simulink model "cobem_simulink_alpha1_0"  (R2018a)
settings: Solver=ode4  StartTime=0.0  StopTime=tempo_simu  FixedStep=1e-3  RelTol=1e-3
values from neighbouring files (symbols this model uses):
  Area1 = 3.1416    [clc.mat]    (also in cobem_teste_PSO.m)
  Area2 = 0.0113    [clc.mat]    (also in cobem_teste_PSO.m)
  Area4 = 0.0314    [clc.mat]    (also in cobem_teste_PSO.m)
  Fnom = 60    [clc.mat]    (also in cobem_teste_PSO.m)
  g = 9.81    [clc.mat]    (also in cobem_teste_PSO.m)
  h10 = 0.5    [clc.mat]    (also in cobem_teste_PSO.m)
  h20 = 0.5    [clc.mat]    (also in cobem_teste_PSO.m)
  Hmax = 3    [clc.mat]    (also in cobem_teste_PSO.m)
  Kd = abs(current_position(3,i))    [cobem_teste_PSO.m]
  Ki = abs(current_position(2,i))    [cobem_teste_PSO.m]
  Kp = abs(current_position(1,i))    [cobem_teste_PSO.m]
  pho = 998.23    [clc.mat]    (also in cobem_teste_PSO.m)
  Qe = 31360.39368    [clc.mat]    (also in cobem_teste_PSO.m)
  Rmax = 1    [clc.mat]    (also in cobem_teste_PSO.m)
  t_filtro = 0.0426    [clc.mat]    (also in cobem_teste_PSO.m)
settings Model: Creator=generic-user  LastModifiedBy=generic-user

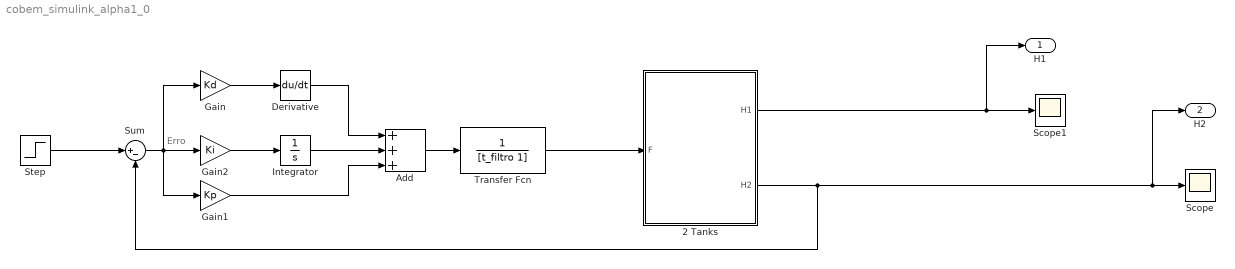
== system cobem_simulink_alpha1_0 ==
  note: Erro
  2 Tanks : Subsystem
  Add : Sum  Inputs=+++
  Derivative : Derivative
  Gain : Gain  Gain=Kd
  Gain1 : Gain  Gain=Kp
  Gain2 : Gain  Gain=Ki
  Integrator : Integrator
  Scope : Scope
  Scope1 : Scope
  Step : Step  Time=0  SampleTime=0
  Sum : Sum  Inputs=|+-
  Transfer Fcn : TransferFcn  Denominator=[t_filtro 1]
  H1 : Outport  SignalName=saida_sys
  H2 : Outport  Port=2  SignalName=saida_sys
  wires:
  2 Tanks/1(H1) -> H1/1, Scope1/1
  2 Tanks/2(H2) -> Sum/2, H2/1, Scope/1
  Step/1 -> Sum/1
  Gain2/1 -> Integrator/1
  Sum/1 -> Gain/1, Gain1/1, Gain2/1
  Gain/1 -> Derivative/1
  Integrator/1 -> Add/2
  Derivative/1 -> Add/1
  Gain1/1 -> Add/3
  Add/1 -> Transfer Fcn/1
  Transfer Fcn/1 -> 2 Tanks/1(F)

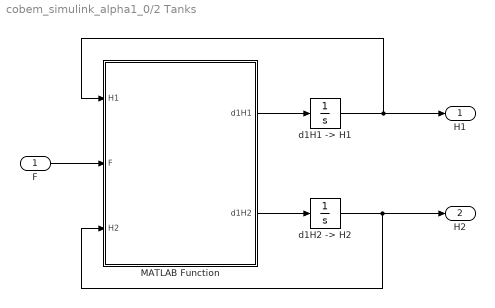
== system cobem_simulink_alpha1_0/2 Tanks ==
  F : Inport
  MATLAB Function : MATLAB Function  TreatAsAtomicUnit=on
  "d1H1 -> H1" : Integrator  InitialCondition=h10  LimitOutput=on  UpperSaturationLimit=10  LowerSaturationLimit=0
  "d1H2 -> H2" : Integrator  InitialCondition=h20  LimitOutput=on  UpperSaturationLimit=10  LowerSaturationLimit=0
  H1 : Outport
  H2 : Outport  Port=2
  wires:
  MATLAB Function/1(d1H1) -> "d1H1 -> H1"/1
  "d1H1 -> H1"/1 -> H1/1, MATLAB Function/1(H1)
  MATLAB Function/2(d1H2) -> "d1H2 -> H2"/1
  F/1 -> MATLAB Function/2(F)
  "d1H2 -> H2"/1 -> H2/1, MATLAB Function/3(H2)

== matlab function cobem_simulink_alpha1_0/2 Tanks/MATLAB Function ==
  data: H1 input; F input; d1H1 output; H2 input; d1H2 output; pho parameter; Fnom parameter; Area1 parameter; Area4 parameter; Hmax parameter; Area2 parameter; g parameter; Qe parameter; Rmax parameter
function [d1H1, d1H2] = TwoTanks(H1, F, H2, pho, Fnom, Area1, Area4, Hmax, Area2, g, Qe, Rmax)

  % Parametros - d1H1
    num1 = Qe;
    den1 = pho*Area1*(Fnom^3);
    num2 = Area2*sqrt(2*g);
    den2 = Area1;
  
  % Parametros - d1H2
    num3 = Area2*sqrt(2*g)*Hmax^2;
    den3 = pi*Rmax^2;
    num4 = Area4*sqrt(2*g)*Hmax^2;
    den4 = pi*Rmax^2;
  
  % Sistema Dinâmico
    d1H1 = (num1/den1)*(F^3) - (num2/den2)*sqrt(H1);
    
    d1H2 = (num3/den3)*(sqrt(H1)/(H2^2)) - (num4/den4)*(1/(H2^1.5));
